simulink model "PCC_Calibration_Simu"  (R2015b)
settings: Solver=ode3  StartTime=0.0  StopTime=1373  FixedStep=0.01  RelTol=1e-3
model workspace: external: MAT-File params.mat (data not in the file)
undefined symbols (not defined in the file): aeroDragCoeff, airDensity, discIntervalf, discIntervals, DiscIntNeverNeededParam, FD, frontArea, G1, G2, G3, G4, G5, G6, gravity, inertialMassVeh, iterNum, lambdaRange, magnitude, massVeh, MDL, powerWeif, powerWeis, predPeriodf, predPeriods, rollingResistCoeff, terminThreshold, terminTimedis, terminVeloweif, terminVeloweis, wheelRadius, z_ACCe
libraries: simulink x16
(part 2 of 5)

== system PCC_Calibration_Simu/Subsystem/vehicle_mode/Glider ==
  note: F_t_r = F_a_e_r_o + F_i + F_g_r_a_d_e + F_r_r
  note: a = (F_t_r - F_a_e_r_o - F_g_r_a_d_e - F_r_r) \div m_i
  note: F_r_r = m g C_r_r
  note: For Analysis & Results
  note: F_a_e_r_o = 1/2 \rho C_d A_f V ^2
  note: F_g_r_a_d_e = m g sin(\theta)
  tractiveForce[N] : Inport
  slope_angle[°] : Inport  Port=2
  AerodynamicDrag[N] : Gain  Gain=0.5*airDensity*aeroDragCoeff*frontArea
      settings: AttributesFormatString=%<Gain>
  AerodynamicDrag[N]1 : Gain  Gain=1.6
      settings: AttributesFormatString=%<Gain>
  Bus Creator : BusCreator  Inputs=7
  Discrete-Time Integrator1 : DiscreteIntegrator  SampleTime=0.01  ICPrevOutput=DiscIntNeverNeededParam  ICPrevScaledInput=DiscIntNeverNeededParam
  Discrete-Time Integrator2 : DiscreteIntegrator  SampleTime=0.01  ICPrevOutput=DiscIntNeverNeededParam  ICPrevScaledInput=DiscIntNeverNeededParam
  Discrete-Time Integrator3 : DiscreteIntegrator  SampleTime=0.01  LimitOutput=on  LowerSaturationLimit=0  ICPrevOutput=DiscIntNeverNeededParam  ICPrevScaledInput=DiscIntNeverNeededParam
  Divide : Product  Inputs=**
  E_brake : Saturate  UpperLimit=0  LowerLimit=-inf
  E_propel : Saturate  UpperLimit=inf  LowerLimit=0
  Force2Acceleration : Gain  Gain=1/inertialMassVeh
      settings: AttributesFormatString=%<Gain>
  GradeForce[N] : Constant  Value=massVeh*gravity
      settings: AttributesFormatString=%<Value>
  J2kWh : Gain  Gain=0.000278/1000
  Product : Product
  RollingResistance[N] : Constant  Value=massVeh*gravity*rollingResistCoeff
      settings: AttributesFormatString=%<Value>
  Sum : Sum  Inputs=+---
  Trigonometric Function : Trigonometry
  Vel^2 : Math  Operator=magnitude^2  SaturateOnIntegerOverflow=on
  mph2mph : Gain  Gain=2.23693629
  veh_spd_acc : Scope
  veh_spd_acc1 : Scope
  veh_spd_acc2 : Scope
  w2kw : Gain  Gain=0.001
  GliderOutput : Outport
  wires:
  J2kWh/1 -> Bus Creator/2  "TotalTractiveEnergy[kWh]"
  Sum/1 -> Force2Acceleration/1, veh_spd_acc1/1  "InertialForce[N]"
  mph2mph/1 -> Bus Creator/6  "Velocity[mph]"
  E_propel/1 -> Bus Creator/4  "PropellingEnergy[J]"
  w2kw/1 -> Bus Creator/1  "TractivePower[kW]"
  Vel^2/1 -> AerodynamicDrag[N]/1
  Discrete-Time Integrator2/1 -> J2kWh/1, Bus Creator/3, E_brake/1, E_propel/1  "TotalTractiveEnergy[J]"
  Force2Acceleration/1 -> Discrete-Time Integrator3/1  "Acceleration[mpss]"
  E_brake/1 -> Bus Creator/5  "BrakingEnergy[J]"
  Discrete-Time Integrator1/1 -> Bus Creator/7  "Position[m]"
  tractiveForce[N]/1 -> Product/1, veh_spd_acc/1, Sum/1  "TractiveForce[N]"
  Product/1 -> Discrete-Time Integrator2/1, w2kw/1  "TractivePower[W]"
  Bus Creator/1 -> GliderOutput/1  "Glider"
  slope_angle[°]/1 -> Trigonometric Function/1
  GradeForce[N]/1 -> Divide/1
  Trigonometric Function/1 -> Divide/2
  Divide/1 -> Sum/4
  RollingResistance[N]/1 -> Sum/3
  AerodynamicDrag[N]/1 -> AerodynamicDrag[N]1/1
  AerodynamicDrag[N]1/1 -> Sum/2
  Discrete-Time Integrator3/1 -> veh_spd_acc2/1, Vel^2/1, Discrete-Time Integrator1/1, Product/2, mph2mph/1  "Velocity[mps]"

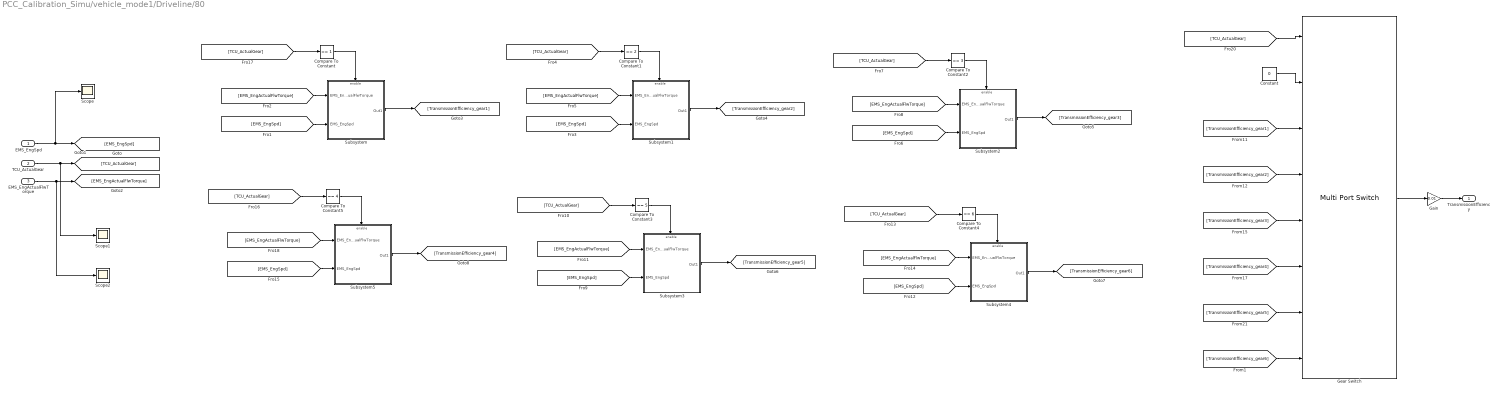
== system PCC_Calibration_Simu/vehicle_mode1/Driveline/80 ==
  EMS_EngSpd : Inport
  TCU_ActualGear : Inport  Port=2
  EMS_EngActualFlwTorque : Inport  Port=3
  Compare To Constant : simulink/Logic and Bit Operations/Compare To Constant  relop===  const=1  OutDataTypeStr=boolean
  Compare To Constant1 : simulink/Logic and Bit Operations/Compare To Constant  relop===  const=2  OutDataTypeStr=boolean
  Compare To Constant2 : simulink/Logic and Bit Operations/Compare To Constant  relop===  const=3  OutDataTypeStr=boolean
  Compare To Constant3 : simulink/Logic and Bit Operations/Compare To Constant  relop===  const=5  OutDataTypeStr=boolean
  Compare To Constant4 : simulink/Logic and Bit Operations/Compare To Constant  relop===  const=6  OutDataTypeStr=boolean
  Compare To Constant5 : simulink/Logic and Bit Operations/Compare To Constant  relop===  const=4  OutDataTypeStr=boolean
  Constant : Constant  Value=0
  Gain : Gain  Gain=0.01
  Gear Switch : MultiPortSwitch  DataPortOrder=Zero-based contiguous  Inputs=7  zeroidx=on
  Scope : Scope
  Scope1 : Scope
  Scope2 : Scope
  Subsystem : Subsystem
  Subsystem1 : Subsystem
  Subsystem2 : Subsystem
  Subsystem3 : Subsystem
  Subsystem4 : Subsystem
  Subsystem5 : Subsystem
  TransmissionEfficiency : Outport
  wires:
  Gain/1 -> TransmissionEfficiency/1
  [TransmissionEfficiency_gear6] -> Gear Switch/8
  Gear Switch/1 -> Gain/1
  [TCU_ActualGear] -> Gear Switch/1
  [TransmissionEfficiency_gear5] -> Gear Switch/7
  [TransmissionEfficiency_gear4] -> Gear Switch/6
  [TransmissionEfficiency_gear3] -> Gear Switch/5
  [TransmissionEfficiency_gear2] -> Gear Switch/4
  [TransmissionEfficiency_gear1] -> Gear Switch/3
  Constant/1 -> Gear Switch/2
  [EMS_EngSpd] -> Subsystem4/2(EMS_EngSpd)
  [EMS_EngActualFlwTorque] -> Subsystem4/1(EMS_EngActualFlwTorque)
  Subsystem4/1(Out1) -> [TransmissionEfficiency_gear6]
  Compare To Constant4/1 -> Subsystem4/Enable
  [TCU_ActualGear] -> Compare To Constant4/1
  [EMS_EngSpd] -> Subsystem3/2(EMS_EngSpd)
  [EMS_EngActualFlwTorque] -> Subsystem3/1(EMS_EngActualFlwTorque)
  Subsystem3/1(Out1) -> [TransmissionEfficiency_gear5]
  Compare To Constant3/1 -> Subsystem3/Enable
  [TCU_ActualGear] -> Compare To Constant3/1
  [EMS_EngSpd] -> Subsystem2/2(EMS_EngSpd)
  [EMS_EngActualFlwTorque] -> Subsystem2/1(EMS_EngActualFlwTorque)
  Subsystem2/1(Out1) -> [TransmissionEfficiency_gear3]
  Compare To Constant2/1 -> Subsystem2/Enable
  [TCU_ActualGear] -> Compare To Constant2/1
  [EMS_EngSpd] -> Subsystem1/2(EMS_EngSpd)
  [EMS_EngActualFlwTorque] -> Subsystem1/1(EMS_EngActualFlwTorque)
  Subsystem1/1(Out1) -> [TransmissionEfficiency_gear2]
  Compare To Constant1/1 -> Subsystem1/Enable
  [TCU_ActualGear] -> Compare To Constant1/1
  [EMS_EngSpd] -> Subsystem5/2(EMS_EngSpd)
  [EMS_EngActualFlwTorque] -> Subsystem5/1(EMS_EngActualFlwTorque)
  Subsystem5/1(Out1) -> [TransmissionEfficiency_gear4]
  Compare To Constant5/1 -> Subsystem5/Enable
  [TCU_ActualGear] -> Compare To Constant5/1
  [EMS_EngSpd] -> Subsystem/2(EMS_EngSpd)
  [EMS_EngActualFlwTorque] -> Subsystem/1(EMS_EngActualFlwTorque)
  Subsystem/1(Out1) -> [TransmissionEfficiency_gear1]
  Compare To Constant/1 -> Subsystem/Enable
  [TCU_ActualGear] -> Compare To Constant/1
  EMS_EngActualFlwTorque/1 -> [EMS_EngActualFlwTorque], Scope2/1
  TCU_ActualGear/1 -> [TCU_ActualGear], Scope1/1
  EMS_EngSpd/1 -> [EMS_EngSpd], Scope/1

== system PCC_Calibration_Simu/vehicle_mode1/Driveline/FindGear ==
  note: Find the current gear based on vehicle speed and driver demand
  APP[%] : Inport
  VehicleSpeed[mph] : Inport  Port=2
  FinalDrive : Gain  Gain=FD
  ShiftLogic : Stateflow chart  TreatAsAtomicUnit=on
  mph2kmph : Gain  Gain=1.609344
  CurrentGear : Outport
  CurrentGearRatio : Outport  Port=2
  wires:
  APP[%]/1 -> ShiftLogic/1(APP)
  mph2kmph/1 -> ShiftLogic/2(VehicleSpeed)
  FinalDrive/1 -> CurrentGearRatio/1
  ShiftLogic/2(GR) -> FinalDrive/1
  ShiftLogic/1(Gear) -> CurrentGear/1
  VehicleSpeed[mph]/1 -> mph2kmph/1

== system PCC_Calibration_Simu/vehicle_mode1/Engine/CalculateEfficiency ==
  EnginePower[W] : Inport
  "EngineSpeed[radps] " : Inport  Port=2
  Constant1 : Constant
  Constant10 : Constant  Value=MDL.EngineModel.C2
  Constant3 : Constant  Value=MDL.EngineModel.EtaT
  Constant6 : Constant  Value=MDL.EngineModel.fmep0
  Constant7 : Constant  Value=MDL.EngineModel.fmep1
  Constant8 : Constant  Value=MDL.EngineModel.Vdisp
  "Divide2  " : Product  Inputs=*/
  MATLAB Function : MATLAB Function  TreatAsAtomicUnit=on
  Switch : Switch  Criteria=u2 > Threshold  ZeroCross=off
  radstorpm : Gain  Gain=9.5488095
  EngineEfficiency : Outport
  wires:
  radstorpm/1 -> MATLAB Function/6(w)
  MATLAB Function/1(eta) -> Switch/1
  [EngSpd] -> radstorpm/1
  Constant10/1 -> MATLAB Function/8(C2)
  Constant8/1 -> MATLAB Function/7(Vdisp)
  Constant7/1 -> MATLAB Function/5(fmep1)
  Constant6/1 -> MATLAB Function/4(fmep0)
  Constant3/1 -> MATLAB Function/3(Etat)
  [EngPwr] -> MATLAB Function/1(Pout)
  Constant1/1 -> Switch/3
  Switch/1 -> EngineEfficiency/1
  EnginePower[W]/1 -> "Divide2  "/1, [EngPwr]
  "Divide2  "/1 -> MATLAB Function/2(Teng), Switch/2  "EngineTorqueOut[Nm]"
  "EngineSpeed[radps] "/1 -> "Divide2  "/2, [EngSpd]

== system PCC_Calibration_Simu/vehicle_mode1/Engine/EnginePower ==
  EngineTorqueOut[Nm] : Inport
  EngineSpeed[radps] : Inport  Port=2
  VehicleSpeed[mph] : Inport  Port=3
  Add : Sum
  Compare To Zero : simulink/Logic and Bit Operations/Compare To Zero  relop=~=  OutDataTypeStr=boolean
  Constant1 : Constant  Value=MDL.EngineModel.AccyLoad
  Ground : Ground
  Memory : Memory
  Product1 : Product  RndMeth=Zero
  Saturation1 : Saturate  UpperLimit=MDL.EngineModel.MaxTrq  LowerLimit=8
  Switch : Switch  Criteria=u2 ~= 0  Threshold=.5
  EnginePowerOutput[W] : Outport
  EngineTorque[Nm] : Outport  Port=2
  wires:
  Compare To Zero/1 -> Switch/2
  Ground/1 -> Switch/3
  EngineTorqueOut[Nm]/1 -> Switch/1
  VehicleSpeed[mph]/1 -> Memory/1
  EngineSpeed[radps]/1 -> Product1/2
  Memory/1 -> Compare To Zero/1
  Product1/1 -> Add/1  "EnginePower[W]"
  Switch/1 -> Saturation1/1  "EngineTorqueOut[Nm]"
  Saturation1/1 -> Product1/1, EngineTorque[Nm]/1
  Add/1 -> EnginePowerOutput[W]/1
  Constant1/1 -> Add/2  "AccessoryLoad[W]"

== system PCC_Calibration_Simu/vehicle_mode1/Engine/EngineTorqueLimiter ==
  note: Find Max Torque Limits
  note: AX7发动机排量为1.997L
  note: 公式为T（Nm）=BMEP(bar)*V(L)/(4*pi*0.01)
  note: 发动机最大功率
  EngineSpeed[radps] : Inport
  1-D Lookup Table : Lookup_n-D  NumberOfTableDimensions=1  BreakpointsForDimension1=[0 1000 1200 1500 1750 2000 2250 2500 2750 3000 3250 3500 3750 4000 4250 4500 4750 5000 5250 5500 5750 6000 6250 6500]  BreakpointsForDimension2=[1:length(MDL.EngineModel.TrqTbl)]  Table=[0 910000 930000 980000 1010000 1050000 1100000 1130000 1100000 1090000 1140000 1170000 1100000 1220000 1200000 1190000 1170000 1150000 1120000 1080000 1040000 1000000 970000 910000]  RndMeth=Simplest  InputSameDT=on
  BMEP2Torque : Gain  Gain=0.001997/(4*pi)
      settings: AttributesFormatString=%<Gain>
  Constant2 : Constant  Value=108000
  Divide2 : Product  Inputs=*/
  MinMax : MinMax  Inputs=2
  radstorpm : Gain  Gain=9.5488095
  MaxEngineTorque[Nm] : Outport
  wires:
  radstorpm/1 -> 1-D Lookup Table/1  "EngineSpeed[rpm]"
  BMEP2Torque/1 -> MinMax/1  "BMEP_LimTorque[Nm]"
  Divide2/1 -> MinMax/2  "PowerLimTorque[Nm]"
  MinMax/1 -> MaxEngineTorque[Nm]/1
  1-D Lookup Table/1 -> BMEP2Torque/1  "BrakeMeanEffectivePressure[Pa]"
  EngineSpeed[radps]/1 -> Divide2/2, radstorpm/1  "EngineSpeed[radps]"
  Constant2/1 -> Divide2/1  "MaxEnginePower[W]"

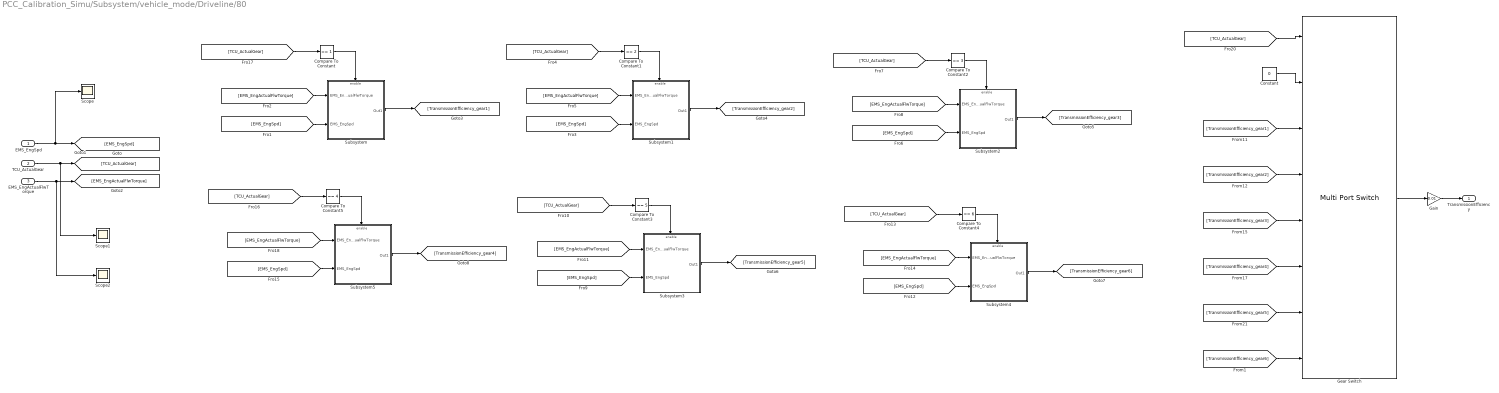
== system PCC_Calibration_Simu/Subsystem/vehicle_mode/Driveline/80 ==
  EMS_EngSpd : Inport
  TCU_ActualGear : Inport  Port=2
  EMS_EngActualFlwTorque : Inport  Port=3
  Compare To Constant : simulink/Logic and Bit Operations/Compare To Constant  relop===  const=1  OutDataTypeStr=boolean
  Compare To Constant1 : simulink/Logic and Bit Operations/Compare To Constant  relop===  const=2  OutDataTypeStr=boolean
  Compare To Constant2 : simulink/Logic and Bit Operations/Compare To Constant  relop===  const=3  OutDataTypeStr=boolean
  Compare To Constant3 : simulink/Logic and Bit Operations/Compare To Constant  relop===  const=5  OutDataTypeStr=boolean
  Compare To Constant4 : simulink/Logic and Bit Operations/Compare To Constant  relop===  const=6  OutDataTypeStr=boolean
  Compare To Constant5 : simulink/Logic and Bit Operations/Compare To Constant  relop===  const=4  OutDataTypeStr=boolean
  Constant : Constant  Value=0
  Gain : Gain  Gain=0.01
  Gear Switch : MultiPortSwitch  DataPortOrder=Zero-based contiguous  Inputs=7  zeroidx=on
  Scope : Scope
  Scope1 : Scope
  Scope2 : Scope
  Subsystem : Subsystem
  Subsystem1 : Subsystem
  Subsystem2 : Subsystem
  Subsystem3 : Subsystem
  Subsystem4 : Subsystem
  Subsystem5 : Subsystem
  TransmissionEfficiency : Outport
  wires:
  EMS_EngSpd/1 -> Scope/1, [EMS_EngSpd]
  TCU_ActualGear/1 -> Scope1/1, [TCU_ActualGear]
  EMS_EngActualFlwTorque/1 -> Scope2/1, [EMS_EngActualFlwTorque]
  [TCU_ActualGear] -> Compare To Constant/1
  Compare To Constant/1 -> Subsystem/Enable
  Subsystem/1(Out1) -> [TransmissionEfficiency_gear1]
  [EMS_EngActualFlwTorque] -> Subsystem/1(EMS_EngActualFlwTorque)
  [EMS_EngSpd] -> Subsystem/2(EMS_EngSpd)
  [TCU_ActualGear] -> Compare To Constant5/1
  Compare To Constant5/1 -> Subsystem5/Enable
  Subsystem5/1(Out1) -> [TransmissionEfficiency_gear4]
  [EMS_EngActualFlwTorque] -> Subsystem5/1(EMS_EngActualFlwTorque)
  [EMS_EngSpd] -> Subsystem5/2(EMS_EngSpd)
  [TCU_ActualGear] -> Compare To Constant1/1
  Compare To Constant1/1 -> Subsystem1/Enable
  Subsystem1/1(Out1) -> [TransmissionEfficiency_gear2]
  [EMS_EngActualFlwTorque] -> Subsystem1/1(EMS_EngActualFlwTorque)
  [EMS_EngSpd] -> Subsystem1/2(EMS_EngSpd)
  [TCU_ActualGear] -> Compare To Constant2/1
  Compare To Constant2/1 -> Subsystem2/Enable
  Subsystem2/1(Out1) -> [TransmissionEfficiency_gear3]
  [EMS_EngActualFlwTorque] -> Subsystem2/1(EMS_EngActualFlwTorque)
  [EMS_EngSpd] -> Subsystem2/2(EMS_EngSpd)
  [TCU_ActualGear] -> Compare To Constant3/1
  Compare To Constant3/1 -> Subsystem3/Enable
  Subsystem3/1(Out1) -> [TransmissionEfficiency_gear5]
  [EMS_EngActualFlwTorque] -> Subsystem3/1(EMS_EngActualFlwTorque)
  [EMS_EngSpd] -> Subsystem3/2(EMS_EngSpd)
  [TCU_ActualGear] -> Compare To Constant4/1
  Compare To Constant4/1 -> Subsystem4/Enable
  Subsystem4/1(Out1) -> [TransmissionEfficiency_gear6]
  [EMS_EngActualFlwTorque] -> Subsystem4/1(EMS_EngActualFlwTorque)
  [EMS_EngSpd] -> Subsystem4/2(EMS_EngSpd)
  Constant/1 -> Gear Switch/2
  [TransmissionEfficiency_gear1] -> Gear Switch/3
  [TransmissionEfficiency_gear2] -> Gear Switch/4
  [TransmissionEfficiency_gear3] -> Gear Switch/5
  [TransmissionEfficiency_gear4] -> Gear Switch/6
  [TransmissionEfficiency_gear5] -> Gear Switch/7
  [TCU_ActualGear] -> Gear Switch/1
  Gear Switch/1 -> Gain/1
  [TransmissionEfficiency_gear6] -> Gear Switch/8
  Gain/1 -> TransmissionEfficiency/1

== system PCC_Calibration_Simu/Subsystem/vehicle_mode/Driveline/FindGear ==
  note: Find the current gear based on vehicle speed and driver demand
  APP[%] : Inport
  VehicleSpeed[mph] : Inport  Port=2
  FinalDrive : Gain  Gain=FD
  ShiftLogic : Stateflow chart  TreatAsAtomicUnit=on
  mph2kmph : Gain  Gain=1.609344
  CurrentGear : Outport
  CurrentGearRatio : Outport  Port=2
  wires:
  VehicleSpeed[mph]/1 -> mph2kmph/1
  ShiftLogic/1(Gear) -> CurrentGear/1
  ShiftLogic/2(GR) -> FinalDrive/1
  FinalDrive/1 -> CurrentGearRatio/1
  mph2kmph/1 -> ShiftLogic/2(VehicleSpeed)
  APP[%]/1 -> ShiftLogic/1(APP)

== system PCC_Calibration_Simu/Subsystem/vehicle_mode/Engine/CalculateEfficiency ==
  EnginePower[W] : Inport
  "EngineSpeed[radps] " : Inport  Port=2
  Constant1 : Constant
  Constant10 : Constant  Value=MDL.EngineModel.C2
  Constant3 : Constant  Value=MDL.EngineModel.EtaT
  Constant6 : Constant  Value=MDL.EngineModel.fmep0
  Constant7 : Constant  Value=MDL.EngineModel.fmep1
  Constant8 : Constant  Value=MDL.EngineModel.Vdisp
  "Divide2  " : Product  Inputs=*/
  MATLAB Function : MATLAB Function  TreatAsAtomicUnit=on
  Switch : Switch  Criteria=u2 > Threshold  ZeroCross=off
  radstorpm : Gain  Gain=9.5488095
  EngineEfficiency : Outport
  wires:
  "EngineSpeed[radps] "/1 -> [EngSpd], "Divide2  "/2
  "Divide2  "/1 -> Switch/2, MATLAB Function/2(Teng)  "EngineTorqueOut[Nm]"
  EnginePower[W]/1 -> [EngPwr], "Divide2  "/1
  Switch/1 -> EngineEfficiency/1
  Constant1/1 -> Switch/3
  [EngPwr] -> MATLAB Function/1(Pout)
  Constant3/1 -> MATLAB Function/3(Etat)
  Constant6/1 -> MATLAB Function/4(fmep0)
  Constant7/1 -> MATLAB Function/5(fmep1)
  Constant8/1 -> MATLAB Function/7(Vdisp)
  Constant10/1 -> MATLAB Function/8(C2)
  [EngSpd] -> radstorpm/1
  MATLAB Function/1(eta) -> Switch/1
  radstorpm/1 -> MATLAB Function/6(w)

== system PCC_Calibration_Simu/Subsystem/vehicle_mode/Engine/EnginePower ==
  EngineTorqueOut[Nm] : Inport
  EngineSpeed[radps] : Inport  Port=2
  VehicleSpeed[mph] : Inport  Port=3
  Add : Sum
  Compare To Zero : simulink/Logic and Bit Operations/Compare To Zero  relop=~=  OutDataTypeStr=boolean
  Constant1 : Constant  Value=MDL.EngineModel.AccyLoad
  Ground : Ground
  Memory : Memory
  Product1 : Product  RndMeth=Zero
  Saturation1 : Saturate  UpperLimit=MDL.EngineModel.MaxTrq  LowerLimit=8
  Switch : Switch  Criteria=u2 ~= 0  Threshold=.5
  EnginePowerOutput[W] : Outport
  EngineTorque[Nm] : Outport  Port=2
  wires:
  Constant1/1 -> Add/2  "AccessoryLoad[W]"
  Add/1 -> EnginePowerOutput[W]/1
  Saturation1/1 -> EngineTorque[Nm]/1, Product1/1
  Switch/1 -> Saturation1/1  "EngineTorqueOut[Nm]"
  Product1/1 -> Add/1  "EnginePower[W]"
  Memory/1 -> Compare To Zero/1
  EngineSpeed[radps]/1 -> Product1/2
  VehicleSpeed[mph]/1 -> Memory/1
  EngineTorqueOut[Nm]/1 -> Switch/1
  Ground/1 -> Switch/3
  Compare To Zero/1 -> Switch/2

== system PCC_Calibration_Simu/Subsystem/vehicle_mode/Engine/EngineTorqueLimiter ==
  note: 发动机最大功率
  note: 公式为T（Nm）=BMEP(bar)*V(L)/(4*pi*0.01)
  note: AX7发动机排量为1.997L
  note: Find Max Torque Limits
  EngineSpeed[radps] : Inport
  1-D Lookup Table : Lookup_n-D  NumberOfTableDimensions=1  BreakpointsForDimension1=[0 1000 1200 1500 1750 2000 2250 2500 2750 3000 3250 3500 3750 4000 4250 4500 4750 5000 5250 5500 5750 6000 6250 6500]  BreakpointsForDimension2=[1:length(MDL.EngineModel.TrqTbl)]  Table=[0 910000 930000 980000 1010000 1050000 1100000 1130000 1100000 1090000 1140000 1170000 1100000 1220000 1200000 1190000 1170000 1150000 1120000 1080000 1040000 1000000 970000 910000]  RndMeth=Simplest  InputSameDT=on
  BMEP2Torque : Gain  Gain=0.001997/(4*pi)
      settings: AttributesFormatString=%<Gain>
  Constant2 : Constant  Value=108000
  Divide2 : Product  Inputs=*/
  MinMax : MinMax  Inputs=2
  radstorpm : Gain  Gain=9.5488095
  MaxEngineTorque[Nm] : Outport
  wires:
  Constant2/1 -> Divide2/1  "MaxEnginePower[W]"
  EngineSpeed[radps]/1 -> radstorpm/1, Divide2/2  "EngineSpeed[radps]"
  1-D Lookup Table/1 -> BMEP2Torque/1  "BrakeMeanEffectivePressure[Pa]"
  MinMax/1 -> MaxEngineTorque[Nm]/1
  Divide2/1 -> MinMax/2  "PowerLimTorque[Nm]"
  BMEP2Torque/1 -> MinMax/1  "BMEP_LimTorque[Nm]"
  radstorpm/1 -> 1-D Lookup Table/1  "EngineSpeed[rpm]"

== system PCC_Calibration_Simu/vehicle_mode1/Driveline/80/Subsystem ==
  EMS_EngActualFlwTorque : Inport
  EMS_EngSpd : Inport  Port=2
  Enable : EnablePort
  2-D Lookup Table : Lookup_n-D  BreakpointsForDimension1=[10 20 25 50 60 75 100 150 200 250]  BreakpointsForDimension2=[750 1000 1500 2000 2500 3000 4000 5000]  Table=[58.5 56.6 52.7 53.5 52.0 50.5 47.7 43.7;74.6 73.7 71.7 74.0 73.4 72.8 72.0 70.0;77.8 77.1 75.5 78.1 77.7 77.2 76.9 75.3;84.3 83.9 83.1 86.3 86.2 86.2 86.6 85.8;85.4 85.0 84.4 87.6 87.6 87.7 88.2 87.6;86.4 86.2 85.7 89.0 89.1 89.1 89.9 89.3;87.5 87.3 86.9 90.4 90.5 90.6 91.5 91.1;88.6 88.4 88.2 91.7 91.9 92.1 93.1 92.8;89.1 89.0 88.8 92.4 92.6 92.9 93.9 93.7;89.4 89.4 89.2 92.8 93.1 93.3 94.4 94.2]  InternalRulePriority=Speed  RndMeth=Simplest  InputSameDT=on
  Out1 : Outport
  wires:
  2-D Lookup Table/1 -> Out1/1
  EMS_EngActualFlwTorque/1 -> 2-D Lookup Table/1
  EMS_EngSpd/1 -> 2-D Lookup Table/2

== system PCC_Calibration_Simu/vehicle_mode1/Driveline/80/Subsystem1 ==
  EMS_EngActualFlwTorque : Inport
  EMS_EngSpd : Inport  Port=2
  Enable : EnablePort
  2-D Lookup Table : Lookup_n-D  BreakpointsForDimension1=[10 20 25 50 60 75 100 150 200 250]  BreakpointsForDimension2=[750 1000 1500 2000 2500 3000 4000 5000]  Table=[61.3 59.2 55.2 53.8 51.4 48.9 46.2 43.0;78.5 77.5 75.6 75.2 73.9 72.6 71.4 69.8;79.9 79.1 77.5 76.9 76.3 75.6 74.7 73.4;86.8 86.4 85.6 85.5 85.3 85.1 84.8 84.1;87.9 87.6 87.0 87.0 86.8 86.7 86.4 85.9;89.1 88.8 88.4 88.4 88.3 88.2 88.1 87.7;90.2 90.0 89.7 89.8 89.8 89.8 89.8 89.5;91.4 91.2 91.1 91.2 91.3 91.4 91.5 91.3;92.0 91.8 91.7 92.0 92.1 92.2 92.3 92.2;92.3 92.2 92.2 92.4 92.5 92.6 92.8 92.7;]  InternalRulePriority=Speed  RndMeth=Simplest  InputSameDT=on
  Out1 : Outport
  wires:
  2-D Lookup Table/1 -> Out1/1
  EMS_EngActualFlwTorque/1 -> 2-D Lookup Table/1
  EMS_EngSpd/1 -> 2-D Lookup Table/2

== system PCC_Calibration_Simu/vehicle_mode1/Driveline/80/Subsystem2 ==
  EMS_EngActualFlwTorque : Inport
  EMS_EngSpd : Inport  Port=2
  Enable : EnablePort
  2-D Lookup Table : Lookup_n-D  BreakpointsForDimension1=[10 20 25 50 60 75 100 150 200 250]  BreakpointsForDimension2=[750 1000 1500 2000 2500 3000 4000 5000]  Table=[63.4 61.1 56.5 54.8 52.6 50.3 46.1 40.7;80.8 79.6 77.3 76.3 75.2 74.0 72.5 69.8;83.7 82.8 81.1 80.3 79.4 78.6 77.4 75.2;89.6 89.2 88.5 88.2 87.9 87.6 87.2 86.1;90.6 90.2 89.7 89.5 89.3 89.1 88.8 87.9;91.6 91.3 91.0 90.8 90.7 90.7 90.4 89.7;92.6 92.4 92.2 92.2 92.2 92.2 92.0 91.5;93.6 93.4 93.4 93.5 93.6 93.7 93.7 93.3;94.1 94.0 94.1 94.1 94.3 94.4 94.5 94.2;94.4 94.3 94.4 94.5 94.7 94.9 95.0 94.8]  InternalRulePriority=Speed  RndMeth=Simplest  InputSameDT=on
  Out1 : Outport
  wires:
  2-D Lookup Table/1 -> Out1/1
  EMS_EngActualFlwTorque/1 -> 2-D Lookup Table/1
  EMS_EngSpd/1 -> 2-D Lookup Table/2

== system PCC_Calibration_Simu/vehicle_mode1/Driveline/80/Subsystem3 ==
  EMS_EngActualFlwTorque : Inport
  EMS_EngSpd : Inport  Port=2
  Enable : EnablePort
  2-D Lookup Table : Lookup_n-D  BreakpointsForDimension1=[10 20 25 50 60 75 100 150 200 250]  BreakpointsForDimension2=[1000 1500 2000 2500 3000 4000 5000 6000]  Table=[48.9 49.2 51.9 49.3 46.8 38.1 29.4 20.7;74.1 74.8 75.7 74.4 73.0 68.3 64.0 59.6;78.5 79.2 80.0 79.0 77.9 74.4 70.9 67.4;87.4 88.1 88.6 88.1 87.6 85.9 84.1 82.4;88.9 89.6 90.0 89.6 89.2 87.6 86.1 84.7;90.2 90.8 91.2 91.0 90.8 89.6 88.5 87.3;91.6 92.1 92.4 92.4 92.3 91.8 91.0 90.1;92.9 93.4 93.5 93.7 93.9 93.9 93.4 92.8;93.6 94.0 94.1 94.4 94.7 94.2 93.8 93.4;93.9 94.4 94.5 94.8 95.1 94.8 94.4 94.1]  InternalRulePriority=Speed  RndMeth=Simplest  InputSameDT=on
  Out1 : Outport
  wires:
  2-D Lookup Table/1 -> Out1/1
  EMS_EngActualFlwTorque/1 -> 2-D Lookup Table/1
  EMS_EngSpd/1 -> 2-D Lookup Table/2

== system PCC_Calibration_Simu/vehicle_mode1/Driveline/80/Subsystem4 ==
  EMS_EngActualFlwTorque : Inport
  EMS_EngSpd : Inport  Port=2
  Enable : EnablePort
  2-D Lookup Table : Lookup_n-D  BreakpointsForDimension1=[10 20 25 50 60 75 100 150 200 250]  BreakpointsForDimension2=[1000 1500 2000 2500 3000 4000 5000 6000]  Table=[39.7 41.1 41.1 36.4 31.8 16.3 0.0 0.0;70.7 70.4 70.4 67.9 65.4 58.1 49.0 40.7;76.0 75.8 75.9 73.9 72.0 66.4 58.8 52.2;86.5 86.6 86.7 85.9 85.2 82.8 78.6 75.3;88.3 88.4 88.5 87.9 87.3 85.5 82.8 80.0;89.6 89.8 90.0 89.5 89.1 87.7 85.5 83.3;90.9 91.3 91.4 91.1 90.8 89.8 88.2 86.5;92.9 93.0 93.1 92.9 92.8 91.9 90.8 89.7;93.9 93.8 93.9 93.8 93.8 93.0 92.2 91.4;94.5 94.4 94.4 94.4 94.3 93.7 93.0 92.3]  InternalRulePriority=Speed  RndMeth=Simplest  InputSameDT=on
  Out1 : Outport
  wires:
  2-D Lookup Table/1 -> Out1/1
  EMS_EngActualFlwTorque/1 -> 2-D Lookup Table/1
  EMS_EngSpd/1 -> 2-D Lookup Table/2

== system PCC_Calibration_Simu/vehicle_mode1/Driveline/80/Subsystem5 ==
  EMS_EngActualFlwTorque : Inport
  EMS_EngSpd : Inport  Port=2
  Enable : EnablePort
  2-D Lookup Table : Lookup_n-D  BreakpointsForDimension1=[10 20 25 50 60 75 100 150 200 250]  BreakpointsForDimension2=[1000 1500 2000 2500 3000 4000 5000 6000]  Table=[45.3 43.8 43.8 39.9 36.0 31.8 27.6 23.4;72.6 71.7 71.7 69.8 67.8 66.3 64.2 62.1;77.4 76.7 76.8 75.3 73.7 72.1 70.4 68.7;86.9 86.6 86.9 86.2 85.6 84.8 83.9 83.1;88.4 88.3 88.6 88.1 87.6 87.3 86.6 85.9;89.9 89.9 90.2 89.8 89.5 88.9 88.4 87.8;91.4 91.5 91.7 91.5 91.4 91.1 90.7 90.3;92.8 93.1 93.3 93.3 93.3 93.0 92.7 92.4;93.5 93.9 94.1 94.2 94.2 94.0 93.8 93.6;94.0 94.3 94.6 94.7 94.8 94.6 94.5 94.3]  InternalRulePriority=Speed  RndMeth=Simplest  InputSameDT=on
  Out1 : Outport
  wires:
  2-D Lookup Table/1 -> Out1/1
  EMS_EngActualFlwTorque/1 -> 2-D Lookup Table/1
  EMS_EngSpd/1 -> 2-D Lookup Table/2

== system PCC_Calibration_Simu/vehicle_mode1/Driveline/FindGear/ShiftLogic/calc_down ==
  Gear : Inport
  APP : Inport  Port=2
  f : TriggerPort  TriggerType=function-call
      settings: CopyFcn=Stateflow.SLINSF.SimulinkMan.removeBlockPreDeleteFcn  PreDeleteFcn=Stateflow.SLINSF.SimulinkMan.unsafePredeleteFcn
  Calculate Downshift Threshold : Lookup2D  RowIndex=PedalPositions  ColumnIndex=[2,3,4,5,6]  Table=DownShiftSpeeds'  LookUpMeth=Interpolation-Use End Values
  down_th : Outport
  wires:
  APP/1 -> Calculate Downshift Threshold/1
  Gear/1 -> Calculate Downshift Threshold/2
  Calculate Downshift Threshold/1 -> down_th/1

== system PCC_Calibration_Simu/vehicle_mode1/Driveline/FindGear/ShiftLogic/calc_up ==
  Gear : Inport
  APP : Inport  Port=2
  f : TriggerPort  TriggerType=function-call
      settings: CopyFcn=Stateflow.SLINSF.SimulinkMan.removeBlockPreDeleteFcn  PreDeleteFcn=Stateflow.SLINSF.SimulinkMan.unsafePredeleteFcn
  Calculate Upshift Threshold : Lookup2D  RowIndex=PedalPositions  ColumnIndex=[1,2,3,4,5]  Table=UpShiftSpeeds'  LookUpMeth=Interpolation-Use End Values
  up_th : Outport
  wires:
  Gear/1 -> Calculate Upshift Threshold/2
  APP/1 -> Calculate Upshift Threshold/1
  Calculate Upshift Threshold/1 -> up_th/1

== system PCC_Calibration_Simu/Subsystem/vehicle_mode/Driveline/80/Subsystem ==
  EMS_EngActualFlwTorque : Inport
  EMS_EngSpd : Inport  Port=2
  Enable : EnablePort
  2-D Lookup Table : Lookup_n-D  BreakpointsForDimension1=[10 20 25 50 60 75 100 150 200 250]  BreakpointsForDimension2=[750 1000 1500 2000 2500 3000 4000 5000]  Table=[58.5 56.6 52.7 53.5 52.0 50.5 47.7 43.7;74.6 73.7 71.7 74.0 73.4 72.8 72.0 70.0;77.8 77.1 75.5 78.1 77.7 77.2 76.9 75.3;84.3 83.9 83.1 86.3 86.2 86.2 86.6 85.8;85.4 85.0 84.4 87.6 87.6 87.7 88.2 87.6;86.4 86.2 85.7 89.0 89.1 89.1 89.9 89.3;87.5 87.3 86.9 90.4 90.5 90.6 91.5 91.1;88.6 88.4 88.2 91.7 91.9 92.1 93.1 92.8;89.1 89.0 88.8 92.4 92.6 92.9 93.9 93.7;89.4 89.4 89.2 92.8 93.1 93.3 94.4 94.2]  InternalRulePriority=Speed  RndMeth=Simplest  InputSameDT=on
  Out1 : Outport
  wires:
  EMS_EngSpd/1 -> 2-D Lookup Table/2
  EMS_EngActualFlwTorque/1 -> 2-D Lookup Table/1
  2-D Lookup Table/1 -> Out1/1

== system PCC_Calibration_Simu/Subsystem/vehicle_mode/Driveline/80/Subsystem1 ==
  EMS_EngActualFlwTorque : Inport
  EMS_EngSpd : Inport  Port=2
  Enable : EnablePort
  2-D Lookup Table : Lookup_n-D  BreakpointsForDimension1=[10 20 25 50 60 75 100 150 200 250]  BreakpointsForDimension2=[750 1000 1500 2000 2500 3000 4000 5000]  Table=[61.3 59.2 55.2 53.8 51.4 48.9 46.2 43.0;78.5 77.5 75.6 75.2 73.9 72.6 71.4 69.8;79.9 79.1 77.5 76.9 76.3 75.6 74.7 73.4;86.8 86.4 85.6 85.5 85.3 85.1 84.8 84.1;87.9 87.6 87.0 87.0 86.8 86.7 86.4 85.9;89.1 88.8 88.4 88.4 88.3 88.2 88.1 87.7;90.2 90.0 89.7 89.8 89.8 89.8 89.8 89.5;91.4 91.2 91.1 91.2 91.3 91.4 91.5 91.3;92.0 91.8 91.7 92.0 92.1 92.2 92.3 92.2;92.3 92.2 92.2 92.4 92.5 92.6 92.8 92.7;]  InternalRulePriority=Speed  RndMeth=Simplest  InputSameDT=on
  Out1 : Outport
  wires:
  EMS_EngSpd/1 -> 2-D Lookup Table/2
  EMS_EngActualFlwTorque/1 -> 2-D Lookup Table/1
  2-D Lookup Table/1 -> Out1/1

== system PCC_Calibration_Simu/Subsystem/vehicle_mode/Driveline/80/Subsystem2 ==
  EMS_EngActualFlwTorque : Inport
  EMS_EngSpd : Inport  Port=2
  Enable : EnablePort
  2-D Lookup Table : Lookup_n-D  BreakpointsForDimension1=[10 20 25 50 60 75 100 150 200 250]  BreakpointsForDimension2=[750 1000 1500 2000 2500 3000 4000 5000]  Table=[63.4 61.1 56.5 54.8 52.6 50.3 46.1 40.7;80.8 79.6 77.3 76.3 75.2 74.0 72.5 69.8;83.7 82.8 81.1 80.3 79.4 78.6 77.4 75.2;89.6 89.2 88.5 88.2 87.9 87.6 87.2 86.1;90.6 90.2 89.7 89.5 89.3 89.1 88.8 87.9;91.6 91.3 91.0 90.8 90.7 90.7 90.4 89.7;92.6 92.4 92.2 92.2 92.2 92.2 92.0 91.5;93.6 93.4 93.4 93.5 93.6 93.7 93.7 93.3;94.1 94.0 94.1 94.1 94.3 94.4 94.5 94.2;94.4 94.3 94.4 94.5 94.7 94.9 95.0 94.8]  InternalRulePriority=Speed  RndMeth=Simplest  InputSameDT=on
  Out1 : Outport
  wires:
  EMS_EngSpd/1 -> 2-D Lookup Table/2
  EMS_EngActualFlwTorque/1 -> 2-D Lookup Table/1
  2-D Lookup Table/1 -> Out1/1

== system PCC_Calibration_Simu/Subsystem/vehicle_mode/Driveline/80/Subsystem3 ==
  EMS_EngActualFlwTorque : Inport
  EMS_EngSpd : Inport  Port=2
  Enable : EnablePort
  2-D Lookup Table : Lookup_n-D  BreakpointsForDimension1=[10 20 25 50 60 75 100 150 200 250]  BreakpointsForDimension2=[1000 1500 2000 2500 3000 4000 5000 6000]  Table=[48.9 49.2 51.9 49.3 46.8 38.1 29.4 20.7;74.1 74.8 75.7 74.4 73.0 68.3 64.0 59.6;78.5 79.2 80.0 79.0 77.9 74.4 70.9 67.4;87.4 88.1 88.6 88.1 87.6 85.9 84.1 82.4;88.9 89.6 90.0 89.6 89.2 87.6 86.1 84.7;90.2 90.8 91.2 91.0 90.8 89.6 88.5 87.3;91.6 92.1 92.4 92.4 92.3 91.8 91.0 90.1;92.9 93.4 93.5 93.7 93.9 93.9 93.4 92.8;93.6 94.0 94.1 94.4 94.7 94.2 93.8 93.4;93.9 94.4 94.5 94.8 95.1 94.8 94.4 94.1]  InternalRulePriority=Speed  RndMeth=Simplest  InputSameDT=on
  Out1 : Outport
  wires:
  EMS_EngSpd/1 -> 2-D Lookup Table/2
  EMS_EngActualFlwTorque/1 -> 2-D Lookup Table/1
  2-D Lookup Table/1 -> Out1/1

== system PCC_Calibration_Simu/Subsystem/vehicle_mode/Driveline/80/Subsystem4 ==
  EMS_EngActualFlwTorque : Inport
  EMS_EngSpd : Inport  Port=2
  Enable : EnablePort
  2-D Lookup Table : Lookup_n-D  BreakpointsForDimension1=[10 20 25 50 60 75 100 150 200 250]  BreakpointsForDimension2=[1000 1500 2000 2500 3000 4000 5000 6000]  Table=[39.7 41.1 41.1 36.4 31.8 16.3 0.0 0.0;70.7 70.4 70.4 67.9 65.4 58.1 49.0 40.7;76.0 75.8 75.9 73.9 72.0 66.4 58.8 52.2;86.5 86.6 86.7 85.9 85.2 82.8 78.6 75.3;88.3 88.4 88.5 87.9 87.3 85.5 82.8 80.0;89.6 89.8 90.0 89.5 89.1 87.7 85.5 83.3;90.9 91.3 91.4 91.1 90.8 89.8 88.2 86.5;92.9 93.0 93.1 92.9 92.8 91.9 90.8 89.7;93.9 93.8 93.9 93.8 93.8 93.0 92.2 91.4;94.5 94.4 94.4 94.4 94.3 93.7 93.0 92.3]  InternalRulePriority=Speed  RndMeth=Simplest  InputSameDT=on
  Out1 : Outport
  wires:
  EMS_EngSpd/1 -> 2-D Lookup Table/2
  EMS_EngActualFlwTorque/1 -> 2-D Lookup Table/1
  2-D Lookup Table/1 -> Out1/1

== system PCC_Calibration_Simu/Subsystem/vehicle_mode/Driveline/80/Subsystem5 ==
  EMS_EngActualFlwTorque : Inport
  EMS_EngSpd : Inport  Port=2
  Enable : EnablePort
  2-D Lookup Table : Lookup_n-D  BreakpointsForDimension1=[10 20 25 50 60 75 100 150 200 250]  BreakpointsForDimension2=[1000 1500 2000 2500 3000 4000 5000 6000]  Table=[45.3 43.8 43.8 39.9 36.0 31.8 27.6 23.4;72.6 71.7 71.7 69.8 67.8 66.3 64.2 62.1;77.4 76.7 76.8 75.3 73.7 72.1 70.4 68.7;86.9 86.6 86.9 86.2 85.6 84.8 83.9 83.1;88.4 88.3 88.6 88.1 87.6 87.3 86.6 85.9;89.9 89.9 90.2 89.8 89.5 88.9 88.4 87.8;91.4 91.5 91.7 91.5 91.4 91.1 90.7 90.3;92.8 93.1 93.3 93.3 93.3 93.0 92.7 92.4;93.5 93.9 94.1 94.2 94.2 94.0 93.8 93.6;94.0 94.3 94.6 94.7 94.8 94.6 94.5 94.3]  InternalRulePriority=Speed  RndMeth=Simplest  InputSameDT=on
  Out1 : Outport
  wires:
  EMS_EngSpd/1 -> 2-D Lookup Table/2
  EMS_EngActualFlwTorque/1 -> 2-D Lookup Table/1
  2-D Lookup Table/1 -> Out1/1

== system PCC_Calibration_Simu/Subsystem/vehicle_mode/Driveline/FindGear/ShiftLogic/calc_down ==
  Gear : Inport
  APP : Inport  Port=2
  f : TriggerPort  TriggerType=function-call
      settings: CopyFcn=Stateflow.SLINSF.SimulinkMan.removeBlockPreDeleteFcn  PreDeleteFcn=Stateflow.SLINSF.SimulinkMan.unsafePredeleteFcn
  Calculate Downshift Threshold : Lookup2D  RowIndex=PedalPositions  ColumnIndex=[2,3,4,5,6]  Table=DownShiftSpeeds'  LookUpMeth=Interpolation-Use End Values
  down_th : Outport
  wires:
  Calculate Downshift Threshold/1 -> down_th/1
  Gear/1 -> Calculate Downshift Threshold/2
  APP/1 -> Calculate Downshift Threshold/1

== system PCC_Calibration_Simu/Subsystem/vehicle_mode/Driveline/FindGear/ShiftLogic/calc_up ==
  Gear : Inport
  APP : Inport  Port=2
  f : TriggerPort  TriggerType=function-call
      settings: CopyFcn=Stateflow.SLINSF.SimulinkMan.removeBlockPreDeleteFcn  PreDeleteFcn=Stateflow.SLINSF.SimulinkMan.unsafePredeleteFcn
  Calculate Upshift Threshold : Lookup2D  RowIndex=PedalPositions  ColumnIndex=[1,2,3,4,5]  Table=UpShiftSpeeds'  LookUpMeth=Interpolation-Use End Values
  up_th : Outport
  wires:
  Calculate Upshift Threshold/1 -> up_th/1
  APP/1 -> Calculate Upshift Threshold/1
  Gear/1 -> Calculate Upshift Threshold/2

== stateflow chart PCC_Calibration_Simu/vehicle_mode1/Driveline/FindGear/ShiftLogic ==
  settings: updateMethod=DISCRETE  sampleTime=0.01
  state gear_state [parallel]
    settings: executionOrder=1
    state first
      entry:
      Gear = 1;
      GR = G1;
    state second
      entry:
      Gear = 2;
      GR = G2;
    state third
      entry:
      Gear = 3;
      GR = G3;
    state fourth
      entry:
      Gear = 4;
      GR = G4;
    state fifth
      entry:
      Gear = 5;
      GR = G5;
    state sixth
      entry:
      Gear = 6;
      GR = G6;
    (default) -> first
    second -> third [order 1] : UP
    first -> second : UP
    fourth -> fifth [order 1] : UP
    fifth -> sixth [order 1] : UP
    third -> fourth [order 1] : UP
    third -> second [order 2] : DOWN
    second -> first [order 2] : DOWN
    fifth -> fourth [order 2] : DOWN
    fourth -> third [order 2] : DOWN
    sixth -> fifth : DOWN
  state selection_state [parallel]
    du:[up_th]=calc_up(Gear,APP);
    du:[down_th]=calc_down(Gear,APP);
    settings: executionOrder=2
    state steady_state
    state upshifting
    state downshifting
    (default) -> steady_state
    steady_state -> upshifting [order 1] : [VehicleSpeed > up_th]
    steady_state -> downshifting [order 2] : [VehicleSpeed < down_th && Gear > 1]
    downshifting -> steady_state [order 2] : [VehicleSpeed > down_th]
    downshifting -> steady_state [order 1] : after(1,tick)
        | [VehicleSpeed <= down_th]
        | {gear_state.DOWN;}
    upshifting -> steady_state [order 1] : after(1,tick)
        | [VehicleSpeed >= up_th]
        | {gear_state.UP;}
    upshifting -> steady_state [order 2] : [VehicleSpeed < up_th]
  state up_th = calc_up(Gear,APP) [function]
  state down_th = calc_down(Gear,APP) [function]
  data: Gear function_input; APP function_input; up_th function_output; Gear function_input; APP function_input; down_th function_output; APP input double [0..100]; VehicleSpeed input double; Gear output double; down_th local double; up_th local double; GR output double; G1 parameter double; G2 parameter double; G3 parameter double; G4 parameter double; G5 parameter double; G6 parameter double
  events: DOWN local EITHER_EDGE_EVENT; UP local EITHER_EDGE_EVENT

== matlab function PCC_Calibration_Simu/vehicle_mode1/Engine/CalculateEfficiency/MATLAB Function ==
  data: Pout input; eta output; Teng input; Etat input; fmep0 input; fmep1 input; w input; Vdisp input; C2 input
function eta = EngineEfficiency(Pout,Teng,Etat,fmep0,fmep1,w,Vdisp,C2)
%#codegen

eta = Pout/(Pout/(Etat/(1+(fmep0+fmep1*w)/(4*pi*Teng/Vdisp)))+C2*Pout^2);

== matlab function PCC_Calibration_Simu/Evalution module/MATLAB Function1 ==
  settings: sampleTime=0.01
  data: y output double; u1 input double; u2 input double; Fuel_ins_map data_store_memory; Fuel_ins_engine_ne data_store_memory; Fuel_ins_engine_te data_store_memory; u3 input; u4 input; u5 input; u6 input; u7 input
function y= fcn(u1,u2,u3,u4,u5,u6,u7)
discIntervalf = u1;
discIntervals = u2;
iterNum = u3;
terminThreshold = u4;
lambdaRange = u5;
predPeriodf = u6;
predPeriods = u7;
A = 23 - (discIntervalf - 0.1)*10 - (discIntervals - 0.1)*10 + (iterNum-20)*0.1 - (terminThreshold-0.2)*10 + (lambdaRange-500)*0.02 + (predPeriodf-7)*0.8 + (predPeriods-15)*0.8;
y=A;
